simulink model "s0512_actualbodyandbankroll_Fr0"  (R2021a)
settings: Solver=FixedStepAuto  StartTime=0.0  StopTime=10.0  RelTol=1e-3
libraries: CarMaker4SL x13
settings Model: Creator=jason  LastModifiedBy=jason

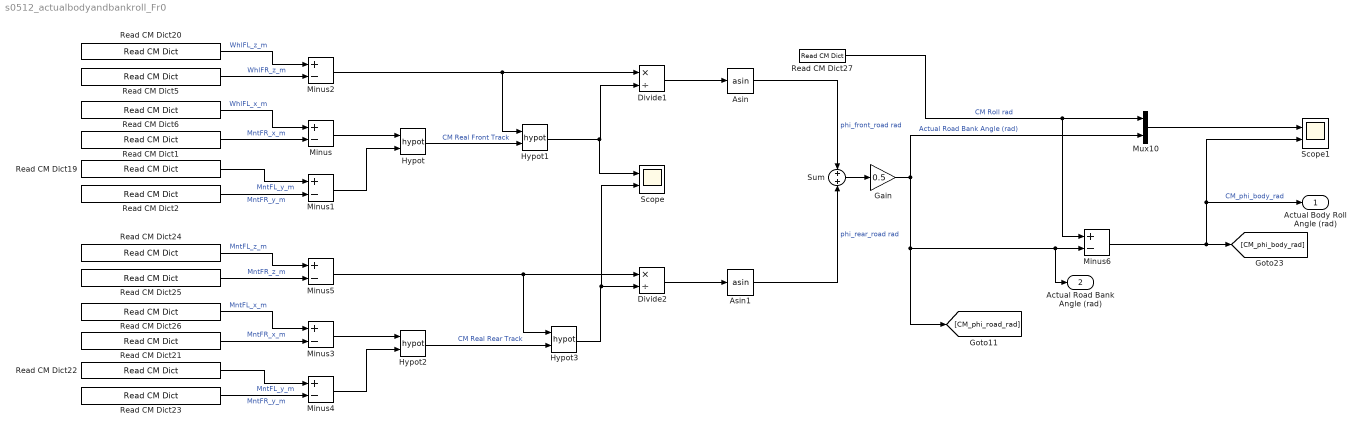
== system s0512_actualbodyandbankroll_Fr0 ==
  Asin : Trigonometry  Operator=asin
  Asin1 : Trigonometry  Operator=asin
  Divide1 : Product  Inputs=*/
  Divide2 : Product  Inputs=*/
  Gain : Gain  Gain=0.5
  Hypot{,1..3} (4 alike) : Math  Operator=hypot  SaturateOnIntegerOverflow=on
  Minus{,1..6} (7 alike) : Sum  Inputs=+-
  Mux10 : Mux  Inputs=2
  Read CM Dict1 : CarMaker4SL/Read CM Dict  xname=Car.CFR.P.t_0.x  xsync=off  xstime=Continuous
  Read CM Dict19 : CarMaker4SL/Read CM Dict  xname=Car.CFL.P.t_0.y  xsync=off  xstime=Continuous
  Read CM Dict2 : CarMaker4SL/Read CM Dict  xname=Car.CFR.P.t_0.y  xsync=off  xstime=Continuous
  Read CM Dict20 : CarMaker4SL/Read CM Dict  xname=Car.CFL.P.t_0.z  xsync=off  xstime=Continuous
  Read CM Dict21 : CarMaker4SL/Read CM Dict  xname=Car.CRR.P.t_0.x  xsync=off  xstime=Continuous
  Read CM Dict22 : CarMaker4SL/Read CM Dict  xname=Car.CRL.P.t_0.y  xsync=off  xstime=Continuous
  Read CM Dict23 : CarMaker4SL/Read CM Dict  xname=Car.CRR.P.t_0.y  xsync=off  xstime=Continuous
  Read CM Dict24 : CarMaker4SL/Read CM Dict  xname=Car.CRL.P.t_0.z  xsync=off  xstime=Continuous
  Read CM Dict25 : CarMaker4SL/Read CM Dict  xname=Car.CRR.P.t_0.z  xsync=off  xstime=Continuous
  Read CM Dict26 : CarMaker4SL/Read CM Dict  xname=Car.CRL.P.t_0.x  xsync=off  xstime=Continuous
  Read CM Dict27 : CarMaker4SL/Read CM Dict  xname=Car.Roll  xsync=off  xstime=Continuous
  Read CM Dict5 : CarMaker4SL/Read CM Dict  xname=Car.CFR.P.t_0.z  xsync=off  xstime=Continuous
  Read CM Dict6 : CarMaker4SL/Read CM Dict  xname=Car.CFL.P.t_0.x  xsync=off  xstime=Continuous
  Scope : Scope  NumInputPorts=2
  Scope1 : Scope  NumInputPorts=2
  Sum : Sum  Inputs=+|+
  Actual Body Roll Angle (rad) : Outport
  Actual Road Bank Angle (rad) : Outport  Port=2
  wires:
  Read CM Dict26/1 -> Minus3/1  "MntFL_x_m"
  Read CM Dict27/1 -> Minus6/1, Mux10/1  "CM Roll rad"
  Minus6/1 -> Actual Body Roll Angle (rad)/1, Scope1/2, [CM_phi_body_rad]  "CM_phi_body_rad"
  Minus5/1 -> Hypot3/1, Divide2/1
  Minus4/1 -> Hypot2/2
  Read CM Dict22/1 -> Minus4/1  "MntFL_y_m"
  Read CM Dict23/1 -> Minus4/2  "MntFR_y_m"
  Mux10/1 -> Scope1/1
  Hypot3/1 -> Scope/2, Divide2/2
  Asin1/1 -> Sum/2  "phi_rear_road rad"
  Hypot1/1 -> Scope/1, Divide1/2
  Sum/1 -> Gain/1
  Read CM Dict1/1 -> Minus/2  "MntFR_x_m"
  Divide2/1 -> Asin1/1
  Read CM Dict25/1 -> Minus5/2  "MntFR_z_m"
  Read CM Dict19/1 -> Minus1/1  "MntFL_y_m"
  Hypot2/1 -> Hypot3/2  "CM Real Rear Track"
  Gain/1 -> Mux10/2, [CM_phi_road_rad], Actual Road Bank Angle (rad)/1, Minus6/2  "Actual Road Bank Angle (rad)"
  Hypot/1 -> Hypot1/2  "CM Real Front Track"
  Read CM Dict20/1 -> Minus2/1  "WhlFL_z_m"
  Read CM Dict24/1 -> Minus5/1  "MntFL_z_m"
  Minus/1 -> Hypot/1
  Asin/1 -> Sum/1  "phi_front_road rad"
  Divide1/1 -> Asin/1
  Minus1/1 -> Hypot/2
  Minus2/1 -> Divide1/1, Hypot1/1
  Read CM Dict5/1 -> Minus2/2  "WhlFR_z_m"
  Minus3/1 -> Hypot2/1
  Read CM Dict6/1 -> Minus/1  "WhlFL_x_m"
  Read CM Dict21/1 -> Minus3/2  "MntFR_x_m"
  Read CM Dict2/1 -> Minus1/2  "MntFR_y_m"
